simulink model "Controlled_Ackermann"  (R2024a)
settings: Solver=VariableStepAuto  StartTime=0.0  StopTime=inf  FixedStep=0.1  MaxStep=0.1  RelTol=1e-3
settings Model: Creator=qiaoyike  LastModifiedBy=qiaoyike
settings RTWCC: GPUComputeCapability=3.5

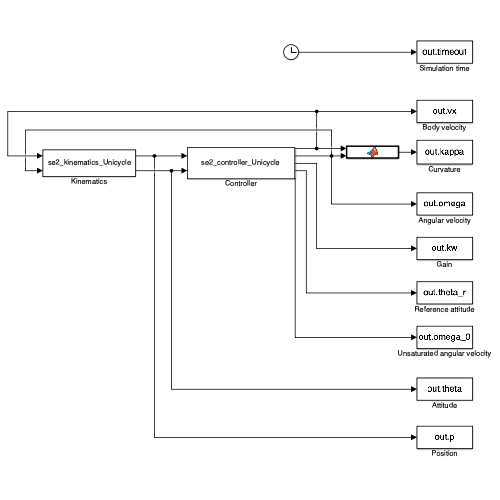
[thumbnail: Simulink's stored preview of the top-level diagram]
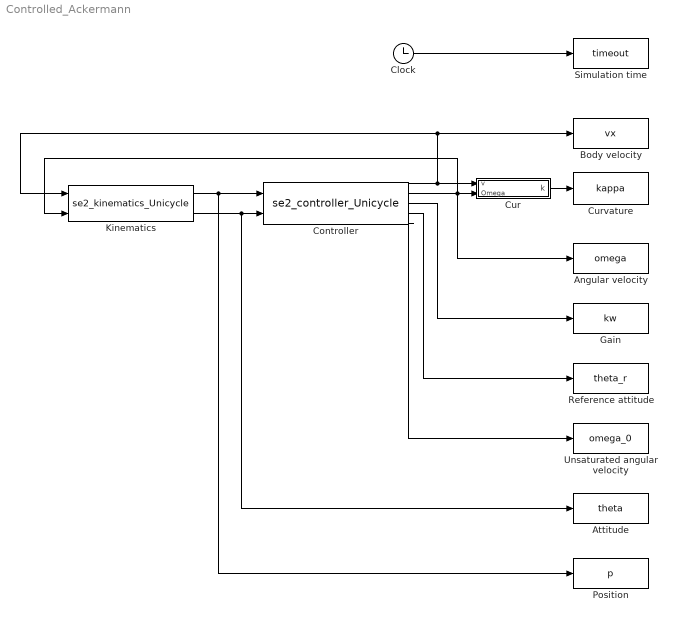
== system Controlled_Ackermann ==
  Angular velocity : ToWorkspace  VariableName=omega  SampleTime=-1
  Attitude : ToWorkspace  VariableName=theta  SampleTime=-1
  Body velocity : ToWorkspace  VariableName=vx  SampleTime=-1
  Clock : Clock
  Controller : M-S-Function  FunctionName=se2_controller_Unicycle  Parameters=p_d,theta_d,rho,v_max,k1,k2,k3  mask{p_d=[4;6.92820323027551], theta_d=2.61799387799149, rho=1, v_max=1, k1=4, k2=8, k3=12}
      mask prompts: p_d "Desired posistion [xd;yd]"; theta_d "Desired orientaion in S"; rho "Minimal turning radius"; v_max "Maximum speed"; k1 "CVF parameters k1"; k2 "CVF parameters k2"; k3 "CVF parameters k3"
      mask DialogControl ParameterGroupVar Prompt: 参数
  Cur : MATLAB Function  TreatAsAtomicUnit=on
  Curvature : ToWorkspace  VariableName=kappa  SampleTime=-1
  Gain : ToWorkspace  VariableName=kw  SampleTime=-1
  Kinematics : M-S-Function  FunctionName=se2_kinematics_Unicycle  Parameters=p_0,theta_0  mask{p_0=[0;0.5], theta_0=3.92699081698724}
      mask prompts: p_0 "Initial position [x0; y0]"; theta_0 "Initial attitude theta_0"
      mask DialogControl ParameterGroupVar Prompt: 参数
  Position : ToWorkspace  VariableName=p  SampleTime=-1
  Reference attitude : ToWorkspace  VariableName=theta_r  SampleTime=-1
  Simulation time : ToWorkspace  VariableName=timeout  SampleTime=-1
  Unsaturated angular velocity : ToWorkspace  VariableName=omega_0  SampleTime=-1
  wires:
  Clock/1 -> Simulation time/1
  Kinematics/1 -> Controller/1, Position/1
  Kinematics/2 -> Controller/2, Attitude/1
  Controller/1 -> Cur/1(v), Kinematics/1, Body velocity/1
  Controller/2 -> Angular velocity/1, Cur/2(Omega), Kinematics/2
  Cur/1(k) -> Curvature/1
  Controller/3 -> Gain/1
  Controller/4 -> Reference attitude/1
  Controller/5 -> Unsaturated angular velocity/1

== matlab function Controlled_Ackermann/Cur ==
  data: v input; k output; Omega input
function k = k(v,Omega)
k = norm(Omega)/norm(v);
